simulink model "ozodo1_m"  (Simulink 7.9)
settings: Solver=ode45  SolverMode=SingleTasking  StartTime=0.0  StopTime=999999  MaxStep=10  RelTol=1e-3  AbsTol=1e-3
values from neighbouring files (symbols this model uses):
  U = st_Varia('LongNames')    [ozodo1_i.m]    (also in ozonox_i.m)
  x0 = []    [ozodo1_i.m]    (also in ozodo1_s.m = x0; ozonox_i.m = [O3*ones(NumCel,1);zeros(NumCel,1);UV254*ones(NumCel,1);zero; ozonox_s.m = x0)
undefined symbols (not defined in the file or in its folder): B
settings Model: Creator=M.Sparnaaij  LastModifiedBy=M.Sparnaaij
settings DataIOCC: LimitDataPoints=off  SaveOutput=off  SaveTime=off  SignalLoggingName=sigsOut
settings OptimizationCC: BooleanDataType=off
settings DebuggingCC: SaveWithParameterizedLinksMsg=none  SignalResolutionControl=TryResolveAllWithWarning  SolverPrmCheckMsg=none  MultiTaskDSMMsg=warning  MultiTaskCondExecSysMsg=none  StrictBusMsg=None
settings HardwareCC: TargetUnknown=on
settings RTWCC: IncludeERTFirstTime=on
settings GRTTargetCC: CombineOutputUpdateFcns=off  GRTInterface=on

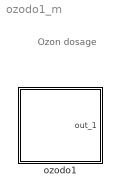
== system ozodo1_m ==
  note: Ozon dosage
  ozodo1 : Subsystem  Description=ozodo1
      mask init:
      | filenaam='.\StimelaData\ozodo1_p.mat';
      | 
      | [Pn,Fn,Fext]=Fileprop(filenaam);
      | 
      | errstr = st_UniqName(filenaam,'filenaam=''','SubSystem','OpenFcn');
      | if errstr, error([errstr 'The filename "' filenaam '" is already in use. Choose a different filename.']), end
      | 
      | P = ozodo1_p(filenaam);
      | [B,x0,U]=ozodo1_i(filenaam);
      settings: OpenFcn=|
      | filenaam='.\StimelaData\ozodo1_p.mat';
      | st_ParameterInput('init',gcb,filenaam,'ozodo1');
      mask Display:
      | plot(0,0,100,100,[90,10],[10,10],[90,10],[30,30],[45,55,55,65,50,35,45,45],[90,90,50,50,30,50,50,90]);
      | disp('')
      | text(50,50,'ozodo1', 'horizontalAlignment', 'center', 'verticalAlignment', 'middle');
      | text(50,0,Fn, 'horizontalAlignment', 'center', 'verticalAlignment', 'base');

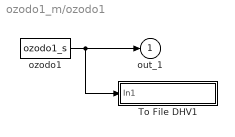
== system ozodo1_m/ozodo1 ==
  To File DHV1 : Subsystem  mask(To File DHV){naam=[filenaam(1:length(filenaam)-4) '_out.sti']}
      mask prompts: naam "Naam van bestand"
      mask init:
      | set_param([gcb '/To File'],'Filename',naam);
      mask Display: disp(naam)
  ozodo1 : S-Function  FunctionName=ozodo1_s  Parameters=B,x0,U,P  EnableBusSupport=off
  out_1 : Outport  InitialOutput=0
  wires:
  ozodo1/1 -> To File DHV1/1(In1), out_1/1

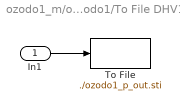
== system ozodo1_m/ozodo1/To File DHV1 ==
  In1 : Inport
  To File : ToFile  Filename=./ozodo1_p_out.sti  MatrixName=ozodo1out
  wires:
  In1/1 -> To File/1
